simulink model "cic2017_boiler_control"  (Simulink 8.3)
settings: Solver=ode23t  StartTime=0.0  StopTime=1000  RelTol=1e-3
undefined symbols (not defined in the file): D0, U0, Y0
settings Model: Creator=Juan  LastModifiedBy=karlos
settings DataIOCC: LimitDataPoints=off
settings OptimizationCC: ExpressionDepthLimit=2147483647  InitFltsAndDblsToZero=on
settings DebuggingCC: SaveWithParameterizedLinksMsg=none  MultiTaskCondExecSysMsg=none  FcnCallInpInsideContextMsg=EnableAllAsWarning
settings SFSimCC: SimParseCustomCode=off
settings RTWCC: IncludeERTFirstTime=on
settings GRTTargetCC: TargetFcnLib=ansi_tfl_tmw.mat

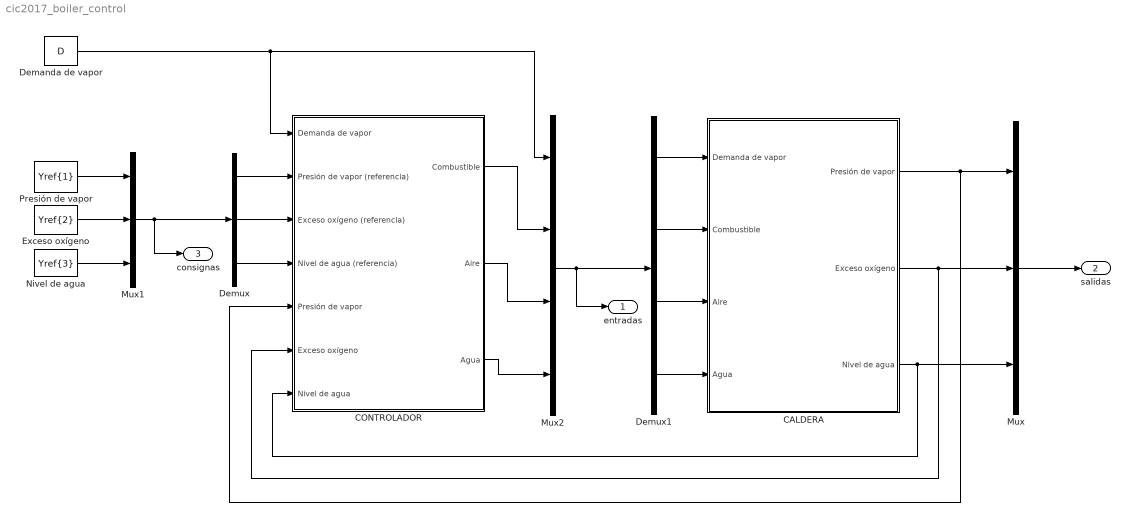
== system cic2017_boiler_control ==
  CALDERA : Subsystem
  CONTROLADOR : Subsystem
  "Demanda de vapor " : FromWorkspace  VariableName=D  SampleTime=0
  Demux : Demux  Outputs=3
  Demux1 : Demux
  Exceso oxígeno : FromWorkspace  VariableName=Yref{2}  SampleTime=0
  Mux : Mux  Inputs=3
  Mux1 : Mux  Inputs=3
  Mux2 : Mux
  Nivel de agua : FromWorkspace  VariableName=Yref{3}  SampleTime=0
  Presión de vapor : FromWorkspace  VariableName=Yref{1}  SampleTime=0
  entradas : Outport
  salidas : Outport  Port=2
  consignas : Outport  Port=3
  wires:
  Mux/1 -> salidas/1
  CALDERA/3(Nivel de agua) -> CONTROLADOR/7(Nivel de agua), Mux/3
  CALDERA/2(Exceso oxígeno) -> CONTROLADOR/6(Exceso oxígeno), Mux/2
  CALDERA/1(Presión de vapor) -> CONTROLADOR/5(Presión de vapor), Mux/1
  Nivel de agua/1 -> Mux1/3
  Exceso oxígeno/1 -> Mux1/2
  Presión de vapor/1 -> Mux1/1
  Mux1/1 -> Demux/1, consignas/1
  Demux/1 -> CONTROLADOR/2(Presión de vapor (referencia))
  Demux/2 -> CONTROLADOR/3(Exceso oxígeno (referencia))
  Demux/3 -> CONTROLADOR/4(Nivel de agua (referencia))
  Mux2/1 -> entradas/1, Demux1/1
  Demux1/3 -> CALDERA/3(Aire)
  Demux1/1 -> CALDERA/1(Demanda de vapor)
  Demux1/2 -> CALDERA/2(Combustible)
  Demux1/4 -> CALDERA/4(Agua)
  "Demanda de vapor "/1 -> Mux2/1, CONTROLADOR/1(Demanda de vapor)
  CONTROLADOR/1(Combustible) -> Mux2/2
  CONTROLADOR/2(Aire) -> Mux2/3
  CONTROLADOR/3(Agua) -> Mux2/4

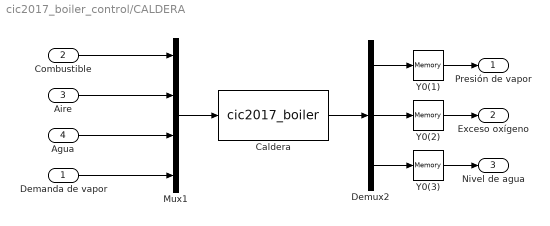
== system cic2017_boiler_control/CALDERA ==
  Demanda de vapor : Inport
  Combustible : Inport  Port=2
  Aire : Inport  Port=3
  Agua : Inport  Port=4
  Caldera : S-Function  FunctionName=cic2017_boiler  Parameters=Y0,[U0 D0]  EnableBusSupport=off
  Demux2 : Demux  Outputs=3
  Mux1 : Mux
  Y0(1) : Memory  X0=Y0(1)
  Y0(2) : Memory  X0=Y0(2)
  Y0(3) : Memory  X0=Y0(3)
  Presión de vapor : Outport
  Exceso oxígeno : Outport  Port=2
  Nivel de agua : Outport  Port=3
  wires:
  Caldera/1 -> Demux2/1
  Aire/1 -> Mux1/2
  Agua/1 -> Mux1/3
  Demanda de vapor/1 -> Mux1/4
  Combustible/1 -> Mux1/1
  Mux1/1 -> Caldera/1
  Demux2/1 -> Y0(1)/1
  Demux2/2 -> Y0(2)/1
  Demux2/3 -> Y0(3)/1
  Y0(1)/1 -> Presión de vapor/1
  Y0(2)/1 -> Exceso oxígeno/1
  Y0(3)/1 -> Nivel de agua/1

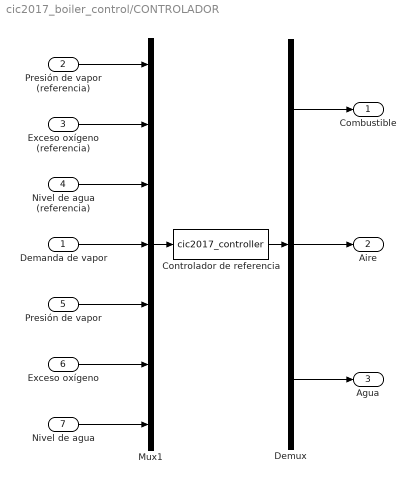
== system cic2017_boiler_control/CONTROLADOR ==
  Demanda de vapor : Inport
  Presión de vapor (referencia) : Inport  Port=2
  Exceso oxígeno (referencia) : Inport  Port=3
  Nivel de agua (referencia) : Inport  Port=4
  Presión de vapor : Inport  Port=5
  Exceso oxígeno : Inport  Port=6
  Nivel de agua : Inport  Port=7
  Controlador de referencia : S-Function  FunctionName=cic2017_controller  EnableBusSupport=off
  Demux : Demux  Outputs=3
  Mux1 : Mux  Inputs=7
  Combustible : Outport
  Aire : Outport  Port=2
  Agua : Outport  Port=3
  wires:
  Nivel de agua/1 -> Mux1/7
  Nivel de agua (referencia)/1 -> Mux1/3
  Demanda de vapor/1 -> Mux1/4
  Presión de vapor/1 -> Mux1/5
  Exceso oxígeno/1 -> Mux1/6
  Exceso oxígeno (referencia)/1 -> Mux1/2
  Presión de vapor (referencia)/1 -> Mux1/1
  Mux1/1 -> Controlador de referencia/1
  Controlador de referencia/1 -> Demux/1
  Demux/1 -> Combustible/1
  Demux/2 -> Aire/1
  Demux/3 -> Agua/1
